simulink model "single_cell_battery"  (R2025b)
settings: Solver=FixedStepDiscrete  StartTime=0.0  StopTime=2000  FixedStep=0.1  RelTol=1e-3
undefined symbols (not defined in the file): C1, C2, DiscIntNeverNeededParam, I_test, ocv_tbl, Q_nom, R0, R1, R2, soc_bp, Ts
settings Model: PacingRate=0.890000  Creator=mahad  LastModifiedBy=mahad
settings DebuggingCC: ReadBeforeWriteMsg=DisableAll  WriteAfterWriteMsg=DisableAll  WriteAfterReadMsg=DisableAll  MultiTaskDSMMsg=none
settings ModelReferenceCC: UpdateModelReferenceTargets=IfOutOfDate
settings SFSimCC: SFSimEcho=off

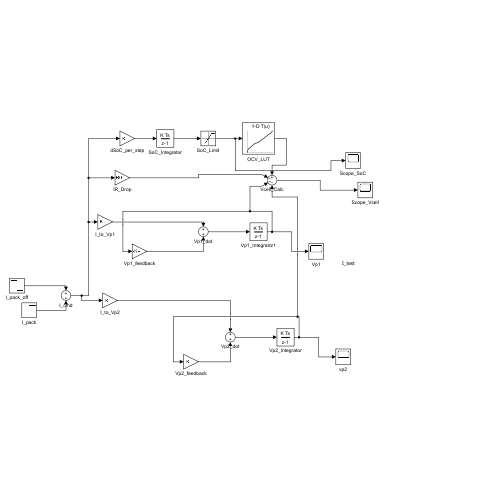
[thumbnail: Simulink's stored preview of the top-level diagram]
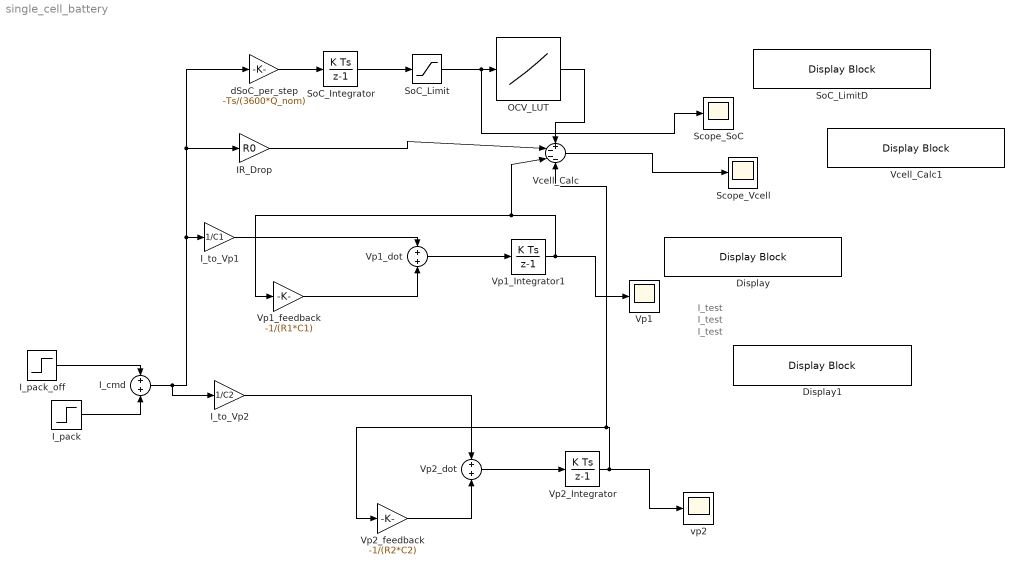
== system single_cell_battery ==
  note: I_test
  note: I_test
  note: I_test
  Display : DisplayBlock  LabelPosition=Hide  Transparency=1  GridColor=[0.502, 0.502, 0.502]
  Display1 : DisplayBlock  LabelPosition=Hide  Transparency=1  GridColor=[0.502, 0.502, 0.502]
  IR_Drop : Gain  Gain=R0
  I_cmd : Sum
  I_pack : Step  After=I_test  SampleTime=0.1
  I_pack_off : Step  Time=20  After=-I_test  SampleTime=0.1
  I_to_Vp1 : Gain  Gain=1/C1
  I_to_Vp2 : Gain  Gain=1/C2
  OCV_LUT : Lookup_n-D  NumberOfTableDimensions=1  BreakpointsForDimension1=soc_bp  Table=ocv_tbl  InternalRulePriority=Speed  RndMeth=Simplest
  Scope_SoC : Scope
  Scope_Vcell : Scope
      settings: ActiveDisplayYMinimum=4.0458316696192469  ActiveDisplayYMaximum=4.101177977939459
  SoC_Integrator : DiscreteIntegrator  InitialCondition=0.95  SampleTime=0.1  ICPrevOutput=DiscIntNeverNeededParam  ICPrevScaledInput=DiscIntNeverNeededParam
  SoC_Limit : Saturate  UpperLimit=1  LowerLimit=0
  SoC_LimitD : DisplayBlock  LabelPosition=Bottom  Transparency=1  GridColor=[0.502, 0.502, 0.502]
  Vcell_Calc : Sum  Inputs=+---
  Vcell_Calc1 : DisplayBlock  LabelPosition=Hide  Transparency=1  GridColor=[0.502, 0.502, 0.502]
  Vp1 : Scope
      settings: ActiveDisplayYMinimum=-0.0017991349349496925  ActiveDisplayYMaximum=0.016192214414547237  DataLoggingVariableName=ScopeData2
  Vp1_Integrator1 : DiscreteIntegrator  SampleTime=0.1  ICPrevOutput=DiscIntNeverNeededParam  ICPrevScaledInput=DiscIntNeverNeededParam
  Vp1_dot : Sum
  Vp1_feedback : Gain  Gain=-1/(R1*C1)
  Vp2_Integrator : DiscreteIntegrator  SampleTime=0.1  ICPrevOutput=DiscIntNeverNeededParam  ICPrevScaledInput=DiscIntNeverNeededParam
  Vp2_dot : Sum
  Vp2_feedback : Gain  Gain=-1/(R2*C2)
  dSoC_per_step : Gain  Gain=-Ts/(3600*Q_nom)
  vp2 : Scope
      settings: ActiveDisplayYMinimum=-0.0017991349349496925  ActiveDisplayYMaximum=0.016192214414547237  DataLoggingVariableName=ScopeData3
  wires:
  dSoC_per_step/1 -> SoC_Integrator/1
  SoC_Integrator/1 -> SoC_Limit/1
  SoC_Limit/1 -> Scope_SoC/1, OCV_LUT/1
  OCV_LUT/1 -> Vcell_Calc/1
  IR_Drop/1 -> Vcell_Calc/2
  Vcell_Calc/1 -> Scope_Vcell/1
  I_to_Vp1/1 -> Vp1_dot/1
  Vp1_Integrator1/1 -> Vp1/1, Vp1_feedback/1, Vcell_Calc/3
  Vp1_dot/1 -> Vp1_Integrator1/1
  Vp1_feedback/1 -> Vp1_dot/2
  Vp2_dot/1 -> Vp2_Integrator/1
  Vp2_Integrator/1 -> vp2/1, Vcell_Calc/4, Vp2_feedback/1
  I_to_Vp2/1 -> Vp2_dot/1
  Vp2_feedback/1 -> Vp2_dot/2
  I_pack_off/1 -> I_cmd/1
  I_pack/1 -> I_cmd/2
  I_cmd/1 -> I_to_Vp2/1, I_to_Vp1/1, IR_Drop/1, dSoC_per_step/1
